simulink model "Double_Tank_sim"  (R2023b)
settings: Solver=VariableStepAuto  StartTime=0.0  StopTime=100  RelTol=1e-3
undefined symbols (not defined in the file): K, V, x_init
libraries: mci_models x2
settings Model: Creator=12064  LastModifiedBy=12064

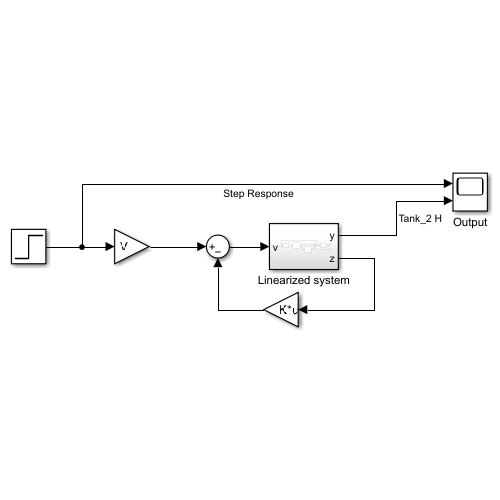
[thumbnail: Simulink's stored preview of the top-level diagram]
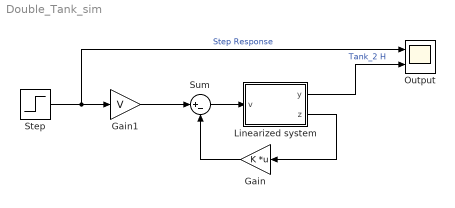
== system Double_Tank_sim ==
  Gain : Gain  Gain=K  Multiplication=Matrix(K*u)
  Gain1 : Gain  Gain=V
  Linearized system : Subsystem
  Output : Scope  NumInputPorts=2
  Step : Step  Time=10  Before=.05  After=.1  SampleTime=0
  Sum : Sum  Inputs=|+-
  wires:
  Linearized system/1(y) -> Output/2  "Tank_2 H"
  Sum/1 -> Linearized system/1(v)
  Linearized system/2(z) -> Gain/1
  Gain/1 -> Sum/2
  Gain1/1 -> Sum/1
  Step/1 -> Output/1, Gain1/1  "Step Response"

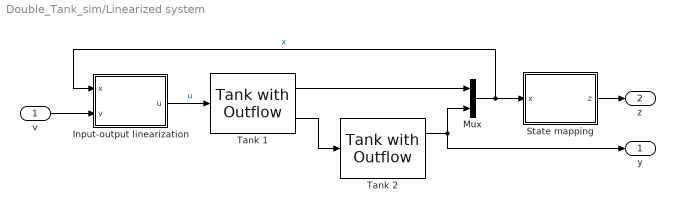
== system Double_Tank_sim/Linearized system ==
  v : Inport
  Input-output linearization : MATLAB Function  TreatAsAtomicUnit=on
  Mux : Mux  Inputs=2
  State mapping : MATLAB Function  TreatAsAtomicUnit=on
  Tank 1 : mci_models/Fluid Systems/Tank with Outflow  At=p.At  Ao=p.Ao  rho=p.rho  zeta=p.zeta  g=9.81  h0=x_init(1)
  Tank 2 : mci_models/Fluid Systems/Tank with Outflow  At=p.At  Ao=p.Ao  rho=p.rho  zeta=p.zeta  g=9.81  h0=x_init(2)
  y : Outport
  z : Outport  Port=2
  wires:
  Tank 1/2 -> Tank 2/1
  Input-output linearization/1(u) -> Tank 1/1  "u"
  v/1 -> Input-output linearization/2(v)
  State mapping/1(z) -> z/1
  Mux/1 -> State mapping/1(x), Input-output linearization/1(x)  "x"
  Tank 1/1 -> Mux/1
  Tank 2/1 -> y/1, Mux/2

== matlab function Double_Tank_sim/Linearized system/Input-output linearization ==
  data: x input; v input; u output; p parameter
function u = fcn(x,v,p)
u = 0;
u = p.rho*p.At*sqrt(x(1))*(2*v/p.a+...
    p.a*sqrt(x(1))/sqrt(x(2)));

== matlab function Double_Tank_sim/Linearized system/State mapping ==
  data: x input; z output; p parameter
function z = fcn(x,p)
%#codegen
z = 0*x; % assignment before subscripting
z(1) = x(2);
z(2) = p.a*sqrt(x(1))-p.a*sqrt(x(2));
